simulink model "Session_1"  (R2023b)
settings: Solver=VariableStepAuto  StartTime=0.0  StopTime=10.0  RelTol=1e-3
undefined symbols (not defined in the file): magnitude
libraries: simulink x2
settings Model: Creator=hp  LastModifiedBy=hp

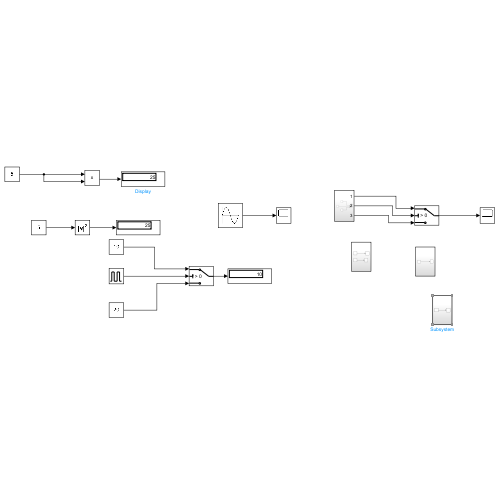
[thumbnail: Simulink's stored preview of the top-level diagram]
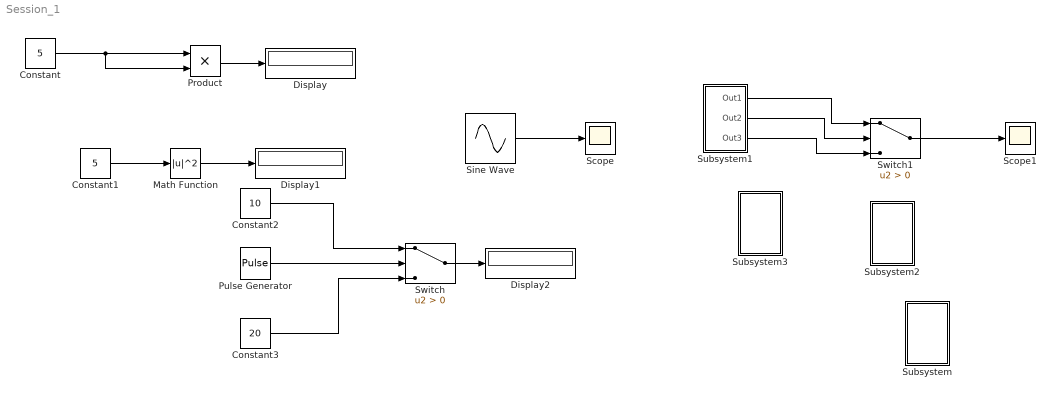
== system Session_1 ==
  Constant : Constant  Value=5
  Constant1 : Constant  Value=5
  Constant2 : Constant  Value=10
  Constant3 : Constant  Value=20
  Display : Display
  Display1 : Display
  Display2 : Display
  Math Function : Math  Operator=magnitude^2
  Product : Product
  Pulse Generator : DiscretePulseGenerator  PulseType=Time based  Period=10  PulseWidth=25
  Scope : Scope
  Scope1 : Scope
  Sine Wave : Sin  Amplitude=10  Frequency=2*pi*2  SampleTime=0
  Subsystem : Subsystem
  Subsystem1 : Subsystem
  Subsystem2 : Subsystem
  Subsystem3 : Subsystem
  Switch : Switch  Criteria=u2 > Threshold  SaturateOnIntegerOverflow=off  InputSameDT=off
  Switch1 : Switch  Criteria=u2 > Threshold  SaturateOnIntegerOverflow=off  InputSameDT=off
  wires:
  Constant/1 -> Product/2, Product/1
  Product/1 -> Display/1
  Constant1/1 -> Math Function/1
  Math Function/1 -> Display1/1
  Sine Wave/1 -> Scope/1
  Constant2/1 -> Switch/1
  Constant3/1 -> Switch/3
  Pulse Generator/1 -> Switch/2
  Switch/1 -> Display2/1
  Switch1/1 -> Scope1/1
  Subsystem1/1(Out1) -> Switch1/1
  Subsystem1/2(Out2) -> Switch1/2
  Subsystem1/3(Out3) -> Switch1/3

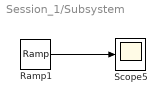
== system Session_1/Subsystem ==
  Ramp1 : simulink/Sources/Ramp  slope=-2  start=0  InitialOutput=5
  Scope5 : Scope
  wires:
  Ramp1/1 -> Scope5/1

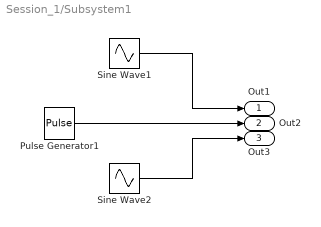
== system Session_1/Subsystem1 ==
  Pulse Generator1 : DiscretePulseGenerator  PulseType=Time based  Period=10  PulseWidth=50
  Sine Wave1 : Sin  SampleTime=0
  Sine Wave2 : Sin  Phase=-pi  SampleTime=0
  Out1 : Outport
  Out2 : Outport  Port=2
  Out3 : Outport  Port=3
  wires:
  Pulse Generator1/1 -> Out2/1
  Sine Wave2/1 -> Out3/1
  Sine Wave1/1 -> Out1/1

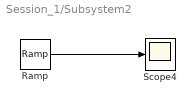
== system Session_1/Subsystem2 ==
  Ramp : simulink/Sources/Ramp  slope=3  start=2  InitialOutput=2
  Scope4 : Scope
  wires:
  Ramp/1 -> Scope4/1

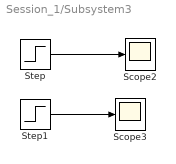
== system Session_1/Subsystem3 ==
  Scope2 : Scope
  Scope3 : Scope
  Step : Step  Time=0  SampleTime=0
  Step1 : Step  Time=0  After=4  SampleTime=0
  wires:
  Step1/1 -> Scope3/1
  Step/1 -> Scope2/1
